simulink subsystem "Scuba_Diver"  (R2026a)
settings: Solver=VariableStepAuto
undefined symbols (not defined in the file): exhale_P_crack
libraries: scuba_lib x13, fl_lib x8, nesl_utility x6
settings Model: Creator=grouleau  LastModifiedBy=grouleau

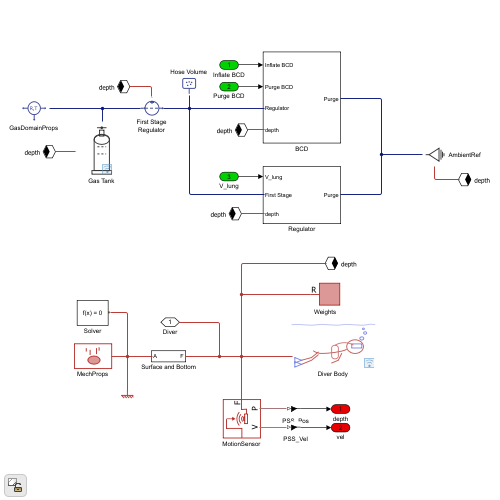
[thumbnail: Simulink's stored preview of the top-level diagram]
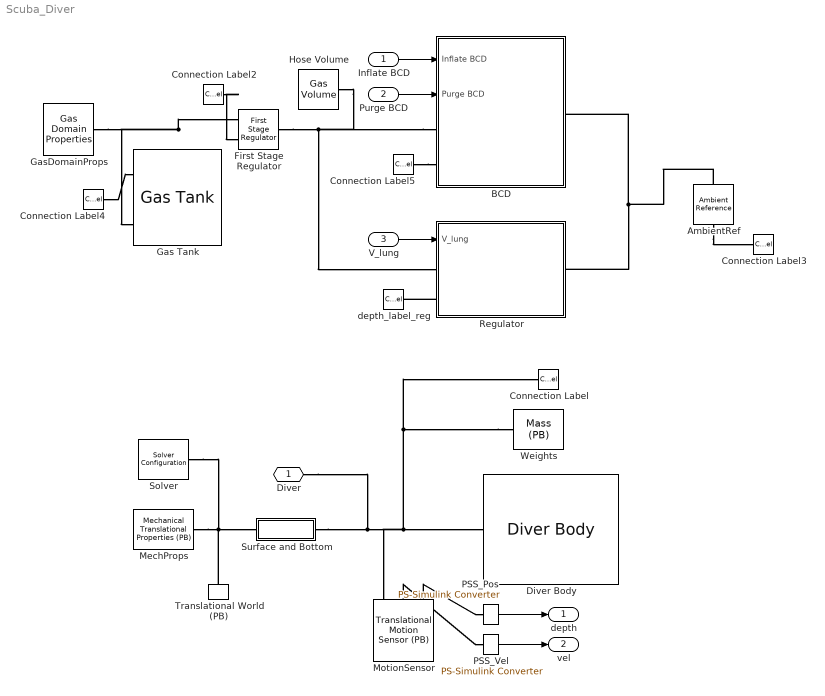
== system Scuba_Diver ==
  Inflate BCD : Inport
  Purge BCD : Inport  Port=2
  V_lung : Inport  Port=3
  AmbientRef : scuba_lib/gas/elements/Ambient Reference  rho_water=1025 kg/m^3  P_atm=101325 Pa  n_dot_in_specify=off  n_dot_in_priority=None  n_dot_in=0 mol/s  n_dot_in_nominal_specify=off  n_dot_in_nominal_value=1  n_dot_in_nominal_unit=mol/s  f_specify=off  f_priority=None  f=0 N  f_nominal_specify=off  f_nominal_value=1  f_nominal_unit=N
  BCD : Subsystem
  Connection Label{,2..5} (5 alike) : ConnectionLabel  Label=depth
  Diver Body : scuba_lib/Diver Body  V_body=0.065 m^3  rho_body=985 kg/m^3  rho_water=1025 kg/m^3  Cd=1.1  A_frontal=0.12 m^2  f_specify=off  f_priority=None  f=0 N  f_nominal_specify=off  f_nominal_value=1  f_nominal_unit=N
  First Stage Regulator : scuba_lib/gas/elements/First Stage Regulator  IP_offset=10e5 Pa  R_open=1e3 Pa*s/mol  rho_water=1025 kg/m^3  P_atm=101325 Pa  n_dot_specify=off  n_dot_priority=None  n_dot=0 mol/s  n_dot_nominal_specify=off  n_dot_nominal_value=1  n_dot_nominal_unit=mol/s  f_specify=off  f_priority=None  f=0 N  f_nominal_specify=off  f_nominal_value=1  f_nominal_unit=N
  Gas Tank : scuba_lib/gas/elements/Gas Tank  V_tank=0.012 m^3  n_init=98.47 mol  M_gas=0.029 kg/mol  n_dot_out_specify=off  n_dot_out_priority=None  n_dot_out=0 mol/s  n_dot_out_nominal_specify=off  n_dot_out_nominal_value=1  n_dot_out_nominal_unit=mol/s  f_specify=off  f_priority=None  f=0 N  f_nominal_specify=off  f_nominal_value=1  f_nominal_unit=N
  GasDomainProps : scuba_lib/gas/elements/Gas Domain Properties  R_gas=8.314 J/(K*mol)  T=293.15 K  n_dot_thru_specify=off  n_dot_thru_priority=None  n_dot_thru=0 mol/s  n_dot_thru_nominal_specify=off  n_dot_thru_nominal_value=1  n_dot_thru_nominal_unit=mol/s
  Hose Volume : scuba_lib/gas/elements/Gas Volume  V=ipvol_V m^3  n_init=ipvol_n_init mol  n_dot_in_specify=off  n_dot_in_priority=None  n_dot_in=0 mol/s  n_dot_in_nominal_specify=off  n_dot_in_nominal_value=1  n_dot_in_nominal_unit=mol/s
  MechProps : fl_lib/Translational/Utilities/Mechanical Translational Properties (PB)  gravity=9.81 m/s^2  beta=-90 deg
  MotionSensor : fl_lib/Translational/Sensors/Translational Motion Sensor (PB)  reference=foundation.enum.MeasurementReference.absolute  acceleration_port=false  velocity_port=true  position_port=true
  PSS_Pos : nesl_utility/PS-Simulink Converter  PhysicalDomain=network_engine_domain  SubClassName=ps_output  LeftPortType=input  RightPortType=output  PseudoPeriodic=off  Frequencies=[]  VectorFormat=inherit  Unit=inherit  AffineConversion=off
  PSS_Vel : nesl_utility/PS-Simulink Converter  PhysicalDomain=network_engine_domain  SubClassName=ps_output  LeftPortType=input  RightPortType=output  PseudoPeriodic=off  Frequencies=[]  VectorFormat=inherit  Unit=inherit  AffineConversion=off
  Regulator : Subsystem
  Solver : nesl_utility/Solver Configuration  PhysicalDomain=network_engine_domain  SubClassName=solver  LeftPortType=input  RightPortType=generic  Tones=[]  Harmonics=[]  SimulateNoise=off  Profile=off  UseLocalSampling=off  EnableSwitchedLinearOptims=on  FrequencyDomain=off  UseCCode=off  RelTol=0.001  AbsTol=0.001  MinStep=1e-09  ToWorkspace=off  RevertToSquareIcSolve=off  NumHomotopyIterations=100  PhasorMode=off  PhasorModeNumHarmonics=1  ConsistencySolver=NEWTON_XTOL_AFTER_FTOL  CanonicalOrdering=CANONICAL  OptimizeIntermediates=OPTIMIZED  IndexReductionMethod=DerivativeReplacement  DoDC=off  ResidualTolerance=1e-09  ConsistencyTolSource=GLOBAL  ConsistencyAbsTol=0.001  ConsistencyRelTol=0.001  ConsistencyTolFactor=0.001  UseLocalSolver=off  LocalSolverChoice=NE_BACKWARD_EULER_ADVANCER  ResolveIndetEquations=on  FunctionEvalNumThread=1  LocalSolverSampleTime=0.001  DoFixedCost=off  MaxNonlinIter=3  MaxModeIter=2  ComputeImpulses=off  ImpulseIterations=2  LinearAlgebra=auto  LinearAlgebraNumThread=0  EquationFormulation=NE_TIME_EF  DelaysMemoryBudget=1024  AutomaticFiltering=on  FilteringTimeConstant=0.001  PartitionStorageMethod=AS_NEEDED  PartitionMemoryBudget=1024  PartitionMethod=ROBUST  MultibodyUseLocalSolver=off  MultibodyLocalSolverChoice=ODE1  MultibodyLocalSolverSampleTime=0.001
  Surface and Bottom : Subsystem
  Translational World (PB) : fl_lib/Translational/Elements/Translational World (PB)
  Weights : fl_lib/Translational/Elements/Mass (PB)  mass=4 kg  v_specify=on  v_priority=High  v=0 m/s  v_nominal_specify=off  v_nominal_value=1  v_nominal_unit=m/s  f_acc_specify=off  f_acc_priority=None  f_acc=0 N  f_acc_nominal_specify=off  f_acc_nominal_value=1  f_acc_nominal_unit=N  f_specify=off  f_priority=None  f=0 N  f_nominal_specify=off  f_nominal_value=1  f_nominal_unit=N
  depth_label_reg : ConnectionLabel  Label=depth
  Diver : PMIOPort  Side=Left
  depth : Outport
  vel : Outport  Port=2
  wires:
  Purge BCD/1 -> BCD/2(Purge BCD)
  Inflate BCD/1 -> BCD/1(Inflate BCD)
  PSS_Vel/1 -> vel/1
  PSS_Pos/1 -> depth/1
  V_lung/1 -> Regulator/1(V_lung)
  connections:
  BCD/RConn1 -- Regulator/RConn1 -- AmbientRef/LConn1
  BCD/LConn1 -- Hose Volume/RConn1 -- First Stage Regulator/RConn1 -- Regulator/LConn1
  GasDomainProps/LConn1 -- First Stage Regulator/LConn1 -- Gas Tank/LConn2
  Weights/LConn1 -- MotionSensor/RConn1 -- Diver Body/LConn1 -- Surface and Bottom/RConn1 -- Diver/RConn1 -- Connection Label/LConn1
  MechProps/RConn1 -- Surface and Bottom/LConn1 -- Translational World (PB)/RConn1 -- Solver/RConn1
  Connection Label5/LConn1 -- BCD/LConn2
  AmbientRef/RConn1 -- Connection Label3/LConn1
  MotionSensor/RConn2 -- PSS_Vel/LConn1
  MotionSensor/RConn3 -- PSS_Pos/LConn1
  Regulator/LConn2 -- depth_label_reg/LConn1
  Connection Label2/LConn1 -- First Stage Regulator/LConn2
  Connection Label4/LConn1 -- Gas Tank/LConn1

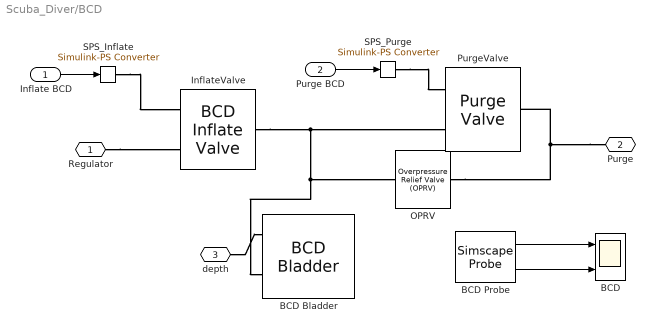
== system Scuba_Diver/BCD ==
  Inflate BCD : Inport
  Purge BCD : Inport  Port=2
  BCD : Scope  NumInputPorts=2
      settings: ActiveDisplayYMinimum=11.711689114793472  ActiveDisplayYMaximum=43.040277393996426  DataLoggingVariableName=ScopeData4
  BCD Bladder : scuba_lib/gas/elements/BCD Bladder  V_max=0.015 m^3  n_init=0.001 mol  K_wall=1e7 Pa/m^3  rho_water=1025 kg/m^3  P_atm=101325 Pa  n_dot_in_specify=off  n_dot_in_priority=None  n_dot_in=0 mol/s  n_dot_in_nominal_specify=off  n_dot_in_nominal_value=1  n_dot_in_nominal_unit=mol/s  f_specify=off  f_priority=None  f=0 N  f_nominal_specify=off  f_nominal_value=1  f_nominal_unit=N  V_bcd_specify=off  V_bcd_priority=None  V_bcd=0 m^3  V_bcd_nominal_specify=off  V_bcd_nominal_value=1  V_bcd_nominal_unit=m^3
  BCD Probe : SimscapeProbe  BoundBlock=6  Variables="{\"A.p\":{\"Unit\":\"psi\",\"Probing\":\"ON\"},\"V_bcd\":{\"Unit\":\"m^3\",\"Probing\":\"ON\"}}"
  InflateValve : scuba_lib/gas/elements/BCD Inflate Valve  R_open=5e6 Pa*s/mol  n_dot_specify=off  n_dot_priority=None  n_dot=0 mol/s  n_dot_nominal_specify=off  n_dot_nominal_value=1  n_dot_nominal_unit=mol/s
  OPRV : scuba_lib/gas/elements/Overpressure Relief Valve (OPRV)  P_crack=20684 Pa  R_open=5000 Pa*s/mol  n_dot_specify=off  n_dot_priority=None  n_dot=0 mol/s  n_dot_nominal_specify=off  n_dot_nominal_value=1  n_dot_nominal_unit=mol/s
  PurgeValve : scuba_lib/gas/elements/Purge Valve  R_open=1e4 Pa*s/mol  P_dump=5000 Pa  n_dot_specify=off  n_dot_priority=None  n_dot=0 mol/s  n_dot_nominal_specify=off  n_dot_nominal_value=1  n_dot_nominal_unit=mol/s
  SPS_Inflate : nesl_utility/Simulink-PS Converter  PhysicalDomain=network_engine_domain  SubClassName=ps_input  LeftPortType=input  RightPortType=output  PseudoPeriodic=off  Frequencies=[]  NoiseDistribution=none  NoiseParameters=[]  Unit=1  AffineConversion=off  FilteringAndDerivatives=provide  SimscapeFilterOrder=1  InputFilterTimeConstant=0.001  UdotUserProvided=0
  SPS_Purge : nesl_utility/Simulink-PS Converter  PhysicalDomain=network_engine_domain  SubClassName=ps_input  LeftPortType=input  RightPortType=output  PseudoPeriodic=off  Frequencies=[]  NoiseDistribution=none  NoiseParameters=[]  Unit=1  AffineConversion=off  FilteringAndDerivatives=provide  SimscapeFilterOrder=1  InputFilterTimeConstant=0.001  UdotUserProvided=0
  Regulator : PMIOPort  Side=Left
  Purge : PMIOPort  Port=2  Side=Right
  depth : PMIOPort  Port=3  Side=Left
  wires:
  BCD Probe/2 -> BCD/2
  BCD Probe/1 -> BCD/1
  Purge BCD/1 -> SPS_Purge/1
  Inflate BCD/1 -> SPS_Inflate/1
  connections:
  Regulator/RConn1 -- InflateValve/LConn1
  SPS_Purge/RConn1 -- PurgeValve/LConn2
  SPS_Inflate/RConn1 -- InflateValve/LConn2
  depth/RConn1 -- BCD Bladder/LConn1
  BCD Bladder/LConn2 -- OPRV/LConn1 -- PurgeValve/LConn1 -- InflateValve/RConn1
  Purge/RConn1 -- PurgeValve/RConn1 -- OPRV/RConn1

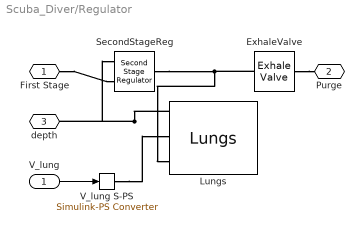
== system Scuba_Diver/Regulator ==
  V_lung : Inport
  ExhaleValve : scuba_lib/gas/elements/Exhale Valve  P_crack=exhale_P_crack*2 Pa  R_open=6000 %exhale_R_open Pa*s/mol  n_dot_specify=off  n_dot_priority=None  n_dot=0 mol/s  n_dot_nominal_specify=off  n_dot_nominal_value=1  n_dot_nominal_unit=mol/s
  Lungs : scuba_lib/gas/elements/Lungs  n_init=lungs_n_init mol  rho_water=1025 kg/m^3  P_atm=101325 Pa  n_dot_specify=off  n_dot_priority=None  n_dot=0 mol/s  n_dot_nominal_specify=off  n_dot_nominal_value=1  n_dot_nominal_unit=mol/s  f_specify=off  f_priority=None  f=0 N  f_nominal_specify=off  f_nominal_value=1  f_nominal_unit=N  P_lung_specify=off  P_lung_priority=None  P_lung=101325 Pa  P_lung_nominal_specify=off  P_lung_nominal_value=1  P_lung_nominal_unit=Pa
  SecondStageReg : scuba_lib/gas/elements/Second Stage Regulator  P_crack=reg2_P_crack Pa  R_open=reg2_R_open Pa*s/mol  rho_water=1025 kg/m^3  P_atm=101325 Pa  n_dot_specify=off  n_dot_priority=None  n_dot=0 mol/s  n_dot_nominal_specify=off  n_dot_nominal_value=1  n_dot_nominal_unit=mol/s  f_specify=off  f_priority=None  f=0 N  f_nominal_specify=off  f_nominal_value=1  f_nominal_unit=N
  V_lung S-PS : nesl_utility/Simulink-PS Converter  PhysicalDomain=network_engine_domain  SubClassName=ps_input  LeftPortType=input  RightPortType=output  PseudoPeriodic=off  Frequencies=[]  NoiseDistribution=none  NoiseParameters=[]  Unit=m^3  AffineConversion=off  FilteringAndDerivatives=filter  SimscapeFilterOrder=2  InputFilterTimeConstant=0.001  UdotUserProvided=0
  First Stage : PMIOPort  Side=Left
  Purge : PMIOPort  Port=2  Side=Right
  depth : PMIOPort  Port=3  Side=Left
  wires:
  V_lung/1 -> V_lung S-PS/1
  connections:
  V_lung S-PS/RConn1 -- Lungs/LConn2
  ExhaleValve/RConn1 -- Purge/RConn1
  Lungs/LConn3 -- ExhaleValve/LConn1 -- SecondStageReg/RConn1
  depth/RConn1 -- SecondStageReg/LConn2 -- Lungs/LConn1
  First Stage/RConn1 -- SecondStageReg/LConn1

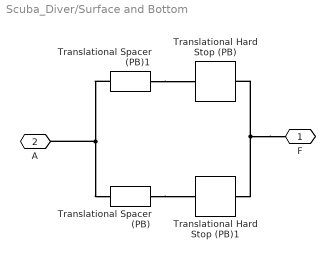
== system Scuba_Diver/Surface and Bottom ==
  Translational Hard Stop (PB) : fl_lib/Translational/Elements/Translational Hard Stop (PB)  model=simscape.enum.hardstop.smooth  stiffness=1e3 N/m  damping=150 N*s/m  transition=0.1 mm  coeff_rest=0.7  initial_state_in_contact=foundation.enum.HardStopInitialState.Free  v_tol=0.001 m/s  f_tol=0.001 N  f_specify=off  f_priority=None  f=0 N  f_nominal_specify=off  f_nominal_value=1  f_nominal_unit=N  v_rel_specify=off  v_rel_priority=None  v_rel=0 m/s  v_rel_nominal_specify=off  v_rel_nominal_value=1  v_rel_nominal_unit=m/s  gap_length_specify=on  gap_length_priority=None  gap_length=0 m  gap_length_nominal_specify=off  gap_length_nominal_value=1  gap_length_nominal_unit=m  length_specify=off  length_priority=None  length=0 m  length_nominal_specify=off  length_nominal_value=1  length_nominal_unit=m
  Translational Hard Stop (PB)1 : fl_lib/Translational/Elements/Translational Hard Stop (PB)  model=simscape.enum.hardstop.smooth  stiffness=1e3 N/m  damping=150 N*s/m  transition=0.1 mm  coeff_rest=0.7  initial_state_in_contact=foundation.enum.HardStopInitialState.Free  v_tol=0.001 m/s  f_tol=0.001 N  f_specify=off  f_priority=None  f=0 N  f_nominal_specify=off  f_nominal_value=1  f_nominal_unit=N  v_rel_specify=off  v_rel_priority=None  v_rel=0 m/s  v_rel_nominal_specify=off  v_rel_nominal_value=1  v_rel_nominal_unit=m/s  gap_length_specify=on  gap_length_priority=None  gap_length=0 m  gap_length_nominal_specify=off  gap_length_nominal_value=1  gap_length_nominal_unit=m  length_specify=off  length_priority=None  length=0 m  length_nominal_specify=off  length_nominal_value=1  length_nominal_unit=m
  Translational Spacer (PB) : fl_lib/Translational/Elements/Translational Spacer (PB)  length_specify=on  length_priority=High  length=50 m  length_nominal_specify=off  length_nominal_value=1  length_nominal_unit=m  f_specify=off  f_priority=None  f=0 N  f_nominal_specify=off  f_nominal_value=1  f_nominal_unit=N
  Translational Spacer (PB)1 : fl_lib/Translational/Elements/Translational Spacer (PB)  length_specify=on  length_priority=High  length=0.1 m  length_nominal_specify=off  length_nominal_value=1  length_nominal_unit=m  f_specify=off  f_priority=None  f=0 N  f_nominal_specify=off  f_nominal_value=1  f_nominal_unit=N
  F : PMIOPort  Side=Right
  A : PMIOPort  Port=2  Side=Left
  connections:
  Translational Spacer (PB)/RConn1 -- Translational Hard Stop (PB)1/RConn1
  Translational Spacer (PB)1/RConn1 -- Translational Hard Stop (PB)/LConn1
  Translational Spacer (PB)/LConn1 -- A/RConn1 -- Translational Spacer (PB)1/LConn1
  F/RConn1 -- Translational Hard Stop (PB)/RConn1 -- Translational Hard Stop (PB)1/LConn1
